simulink model "Z_Feedback"  (R2022b)
settings: Solver=FixedStepAuto  StartTime=0.0  StopTime=10.0  FixedStep=step_size  RelTol=1e-3
undefined symbols (not defined in the file): K_d, K_p, theta_i, x_i, y_i
libraries: simulink_extras x1
settings Model: Creator=Musta  LastModifiedBy=Musta

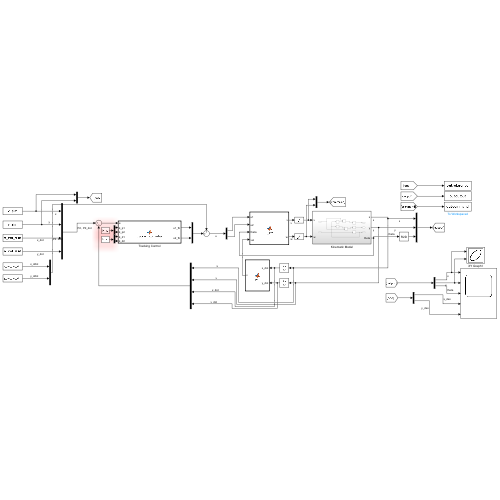
[thumbnail: Simulink's stored preview of the top-level diagram]
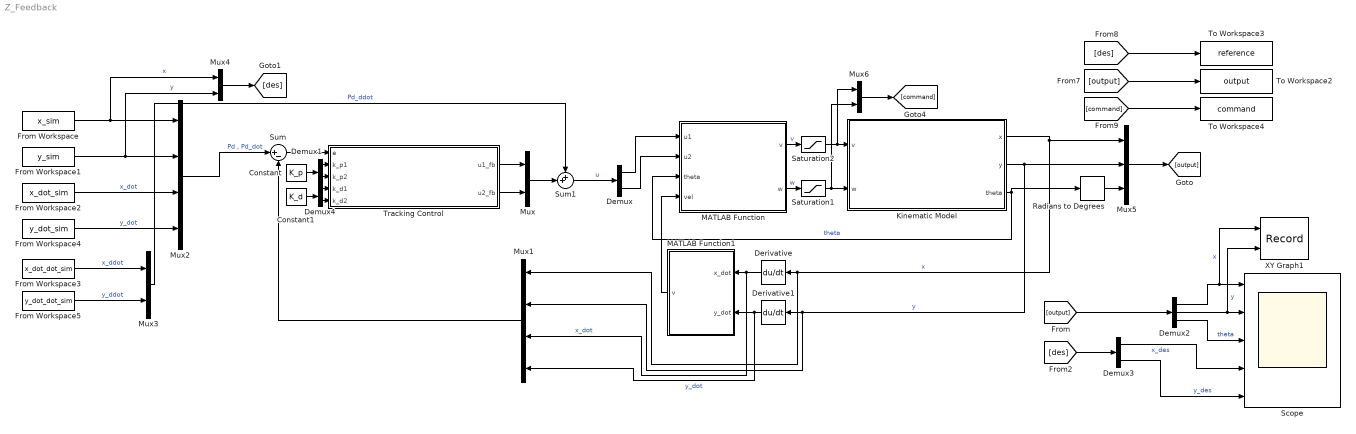
== system Z_Feedback ==
  Constant : Constant  Value=K_p
  Constant1 : Constant  Value=K_d
  Demux{,1,3..4} (4 alike) : Demux  Outputs=2
  Demux2 : Demux  Outputs=3
  Derivative : Derivative
  Derivative1 : Derivative
  From Workspace : FromWorkspace  VariableName=x_sim
  From Workspace1 : FromWorkspace  VariableName=y_sim
  From Workspace2 : FromWorkspace  VariableName=x_dot_sim
  From Workspace3 : FromWorkspace  VariableName=x_dot_dot_sim
  From Workspace4 : FromWorkspace  VariableName=y_dot_sim
  From Workspace5 : FromWorkspace  VariableName=y_dot_dot_sim
  Kinematic Model : Subsystem
  MATLAB Function : MATLAB Function  TreatAsAtomicUnit=on
  MATLAB Function1 : MATLAB Function  TreatAsAtomicUnit=on
  Mux{,3..4,6} (4 alike) : Mux  Inputs=2
  Mux1 : Mux
  Mux2 : Mux
  Mux5 : Mux  Inputs=3
  Radians to Degrees : simulink_extras/Transformations/Radians to Degrees
  Saturation1 : Saturate  UpperLimit=2  LowerLimit=-2
  Saturation2 : Saturate  UpperLimit=2  LowerLimit=-2
  Scope : Scope  NumInputPorts=5
  Sum : Sum  Inputs=|+-
  Sum1 : Sum  Inputs=++|
  To Workspace2 : ToWorkspace  VariableName=output  SaveFormat=Structure With Time  SampleTime=-1
  To Workspace3 : ToWorkspace  VariableName=reference  SaveFormat=Structure With Time  SampleTime=-1
  To Workspace4 : ToWorkspace  VariableName=command  SaveFormat=Structure With Time  SampleTime=-1
  Tracking Control : MATLAB Function  TreatAsAtomicUnit=on
  XY Graph1 : Record  FileSettingsInternal="{\"entries\":[{\"content\":{\"excelSettings\":{\"content\":{},\"type\":\"Streamout.ExcelSettings\"}},\"type\":\"Streamout.FileSettingStorage\",\"uuid\":\"a8dc78ea-e018-43ee-9ce6-9f039c81d0b7\"}],\"packageUris\":[\"http://schema.mathworks.com/mf0/streamout_blocks/R2020a\"],\"version\":\"1.0\"}"  Layout=[1 1]  SignalsInternal="{\"entries\":[{\"content\":{\"signals\":[{\"content\":{\"blockPath\":[\"Z_Feedback_MATLAB/XY Graph1\"],\"channel\":[],\"dimensions\":[1],\"domain\":\"Z_Feedback_MATLAB/XY Graph1\",\"lineColor\":\"#a2142f\",\"plots\":[1],\"port\":1,\"sid\":[\"\"],\"signalID\":915,\"signalName\":\"x\"},\"type\":\"RecordBlkView.Signal\",\"uuid\":\"f428528e-22f6-48e8-82b2-ec440df36d04\"},{\"content\":{\"blockPath\":[\"Z_Feedback_MATLAB/XY Graph1\"],\"channel\":[],\"dimensions\":[1],\"domain\":\"Z_Feedback_MATLAB/XY Graph1\",\"lineColor\":\"#139fff\",\"plots\":[1],\"port\":2,\"sid\":[\"\"],\"signalID\":919,\"signalName\":\"y\"},\"type\":\"RecordBlkView.Signal\",\"uuid\":\"ffbe675b-ad58-4192-96c5-7d702f565157\"}]},\"type\":\"RecordBlkView.InputSignals\",\"uuid\":\"92750eab-5794-4c82-8be6-ab64c90d2cad\"}],\"packageUris\":[\"http://schema.mathworks.com/mf0/streamout_blocks/R2020a\"],\"version\":\"1.0\"}"  VisualizationBindings="{\"xyplotplugin\":{\"info\":[{\"series\":[{\"bindingParametersList\":[{\"parameter\":\"X-Axis\",\"signalID\":915,\"signalName\":\"x\"},{\"parameter\":\"Y-Axis\",\"signalID\":919,\"signalName\":\"y\"}],\"seriesID\":40585}],\"subplotID\":1}]}}"  CompatibilityTag=XY
  wires:
  Saturation1/1 -> Mux6/2, Kinematic Model/2(w)
  Saturation2/1 -> Mux6/1, Kinematic Model/1(v)
  Mux4/1 -> [des]
  Mux1/1 -> Sum/2
  Kinematic Model/1(x) -> Mux5/1, Mux1/1, Derivative/1  "x"
  Mux2/1 -> Sum/1  "Pd , Pd_dot"
  Radians to Degrees/1 -> Mux5/3
  [des] -> Demux3/1
  Kinematic Model/3(theta) -> Radians to Degrees/1, MATLAB Function/3(theta)  "theta"
  Demux3/1 -> Scope/4  "x_des"
  Demux/1 -> MATLAB Function/1(u1)
  Mux/1 -> Sum1/2
  Derivative1/1 -> MATLAB Function1/2(y_dot), Mux1/4  "y_dot"
  From Workspace5/1 -> Mux3/2  "y_ddot"
  Derivative/1 -> Mux1/3, MATLAB Function1/1(x_dot)  "x_dot"
  Demux/2 -> MATLAB Function/2(u2)
  Tracking Control/2(u2_fb) -> Mux/2
  From Workspace1/1 -> Mux2/2, Mux4/2  "y"
  [output] -> To Workspace2/1
  MATLAB Function1/1(v) -> MATLAB Function/4(vel)
  From Workspace3/1 -> Mux3/1  "x_ddot"
  Mux6/1 -> [command]
  [output] -> Demux2/1
  Tracking Control/1(u1_fb) -> Mux/1
  MATLAB Function/1(v) -> Saturation2/1  "v"
  Sum1/1 -> Demux/1  "u"
  MATLAB Function/2(w) -> Saturation1/1  "w"
  Sum/1 -> Tracking Control/1(e)
  Demux2/2 -> XY Graph1/2, Scope/2  "y"
  Kinematic Model/2(y) -> Mux1/2, Derivative1/1, Mux5/2  "y"
  Mux5/1 -> [output]
  Demux3/2 -> Scope/5  "y_des"
  From Workspace/1 -> Mux4/1, Mux2/1  "x"
  [des] -> To Workspace3/1
  From Workspace2/1 -> Mux2/3  "x_dot"
  From Workspace4/1 -> Mux2/4  "y_dot"
  Demux2/1 -> XY Graph1/1, Scope/1  "x"
  Demux2/3 -> Scope/3  "theta"
  [command] -> To Workspace4/1
  Mux3/1 -> Sum1/1  "Pd_ddot"
  Constant/1 -> Demux1/1
  Demux1/1 -> Tracking Control/2(k_p1)
  Demux1/2 -> Tracking Control/3(k_p2)
  Demux4/2 -> Tracking Control/5(k_d2)
  Constant1/1 -> Demux4/1
  Demux4/1 -> Tracking Control/4(k_d1)

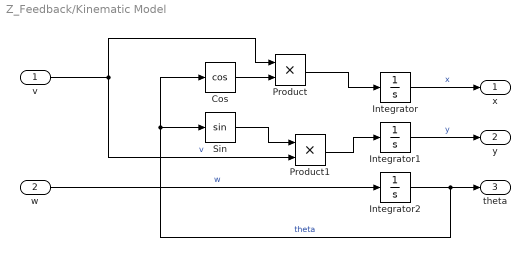
== system Z_Feedback/Kinematic Model ==
  v : Inport
  w : Inport  Port=2
  Cos : Trigonometry  Operator=cos
  Integrator : Integrator  InitialCondition=x_i
  Integrator1 : Integrator  InitialCondition=y_i
  Integrator2 : Integrator  InitialCondition=theta_i
  Product : Product
  Product1 : Product
  Sin : Trigonometry
  x : Outport
  y : Outport  Port=2
  theta : Outport  Port=3
  wires:
  Cos/1 -> Product/2
  Integrator/1 -> x/1  "x"
  Integrator2/1 -> Cos/1, Sin/1, theta/1  "theta"
  Product1/1 -> Integrator1/1
  w/1 -> Integrator2/1  "w"
  Product/1 -> Integrator/1
  v/1 -> Product/1, Product1/2  "v"
  Sin/1 -> Product1/1
  Integrator1/1 -> y/1  "y"

== matlab function Z_Feedback/MATLAB Function ==
  data: u1 input; u2 input; theta input; v output; w output; vel input
function [v,w] = T_inv(u1,u2,theta,vel)


if abs(vel) < 1e-3
    if abs(vel) >= 0
        vel = 1e-3;
    else 
        vel = -1e-3;
    end
end

T_i = [cos(theta) sin(theta);
      -sin(theta)/vel cos(theta)/vel];

v_w = T_i * [u1;u2];

v = v_w(1);
w = v_w(2);

== matlab function Z_Feedback/Tracking Control ==
  data: u1_fb output; u2_fb output; e input; k_p1 input; k_p2 input; k_d1 input; k_d2 input
function [u1_fb,u2_fb] = tracking_controller(e, k_p1, k_p2, k_d1, k_d2)

    e_x = e(1);
    e_y = e(2);
    e_xdot = e(3);
    e_ydot = e(4);
    
    % Controller
    u1_fb = k_p1 * e_x + k_d1 * e_xdot;
    u2_fb = k_p2 *e_y + k_d2 * e_ydot;

end

== matlab function Z_Feedback/MATLAB Function1 ==
  data: x_dot input; v output; y_dot input
function v = vel(x_dot,y_dot)

v = sqrt(x_dot^2 + y_dot^2);
